simulink model "GMSK"  (R2015b)
settings: Solver=ode45  StartTime=0.0  StopTime=1000  RelTol=1e-3
undefined symbols (not defined in the file or in its folder): i
libraries: commdigbbndcpm2 x1, commrandsrc2 x1, commutil2 x1
settings Model: Creator=Алексей  LastModifiedBy=Sam
settings DataIOCC: SaveFormat=Array
settings HardwareCC: ProdBitPerPointer=32  ProdLargestAtomicFloat=None  ProdIntDivRoundTo=Undefined  ProdEndianess=Unspecified  ProdWordSize=32  ProdHWDeviceType=32-bit Generic
settings GRTTargetCC: GeneratePreprocessorConditionals=Disable all
settings ConfigComp: CovModelRefEnable=Off

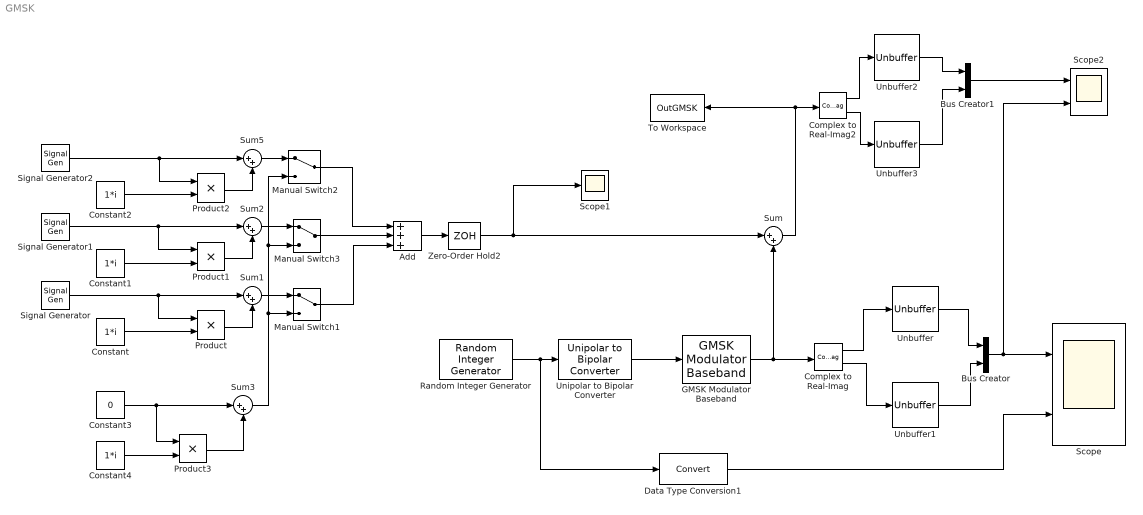
== system GMSK ==
  Add : Sum  Inputs=+++
  Bus Creator : BusCreator  Inputs=2
  Bus Creator1 : BusCreator  Inputs=2
  Complex to Real-Imag : ComplexToRealImag
  Complex to Real-Imag2 : ComplexToRealImag
  Constant{,1..2,4} (4 alike) : Constant  Value=1*i
  Constant3 : Constant  Value=0
  Data Type Conversion1 : DataTypeConversion
  GMSK Modulator Baseband : commdigbbndcpm2/GMSK Modulator Baseband  inputType=Integer  BT=.3  pulseLength=4  preHistory=1  phaseOffset=0  samplesPerSymbol=8  RateOptions=Enforce single-rate processing  outDataType=double
  Manual Switch1 : ManualSwitch
  Manual Switch2 : ManualSwitch
  Manual Switch3 : ManualSwitch
  Product{,1..3} (4 alike) : Product
  Random Integer Generator : commrandsrc2/Random Integer Generator  mul=2  seed=37  Ts=1  frameBased=off  sampPerFrame=1  orient=off  outDataType=boolean
  Scope : Scope  NumInputPorts=2
  Scope1 : Scope
  Scope2 : Scope  NumInputPorts=2
  Signal Generator : SignalGenerator  Amplitude=0.3  Frequency=100  Units=rad/sec
  Signal Generator1 : SignalGenerator  Amplitude=0.35  Frequency=1000  Units=rad/sec
  Signal Generator2 : SignalGenerator  Amplitude=0.5  Frequency=500  Units=rad/sec
  Sum{,1..3,5} (5 alike) : Sum  Inputs=|++
  To Workspace : ToWorkspace  VariableName=OutGMSK  SaveFormat=Timeseries  SampleTime=-1
      settings: Save2DSignal=2-D array (concatenate along first dimension)
  Unbuffer{,1..3} (4 alike) : Unbuffer  SampleBasedProcessing=Same as frame based
  Unipolar to Bipolar Converter : commutil2/Unipolar to Bipolar Converter  M=2  polarity=Positive  dataType=Inherit via internal rule
  Zero-Order Hold2 : ZeroOrderHold
  wires:
  Unipolar to Bipolar Converter/1 -> GMSK Modulator Baseband/1
  GMSK Modulator Baseband/1 -> Complex to Real-Imag/1, Sum/2
  Complex to Real-Imag/1 -> Unbuffer/1
  Complex to Real-Imag/2 -> Unbuffer1/1
  Unbuffer/1 -> Bus Creator/1
  Random Integer Generator/1 -> Data Type Conversion1/1, Unipolar to Bipolar Converter/1
  Bus Creator/1 -> Scope2/2, Scope/1
  Data Type Conversion1/1 -> Scope/2
  Unbuffer1/1 -> Bus Creator/2
  Signal Generator/1 -> Product/1, Sum1/1
  Complex to Real-Imag2/2 -> Unbuffer3/1
  Complex to Real-Imag2/1 -> Unbuffer2/1
  Bus Creator1/1 -> Scope2/1
  Unbuffer2/1 -> Bus Creator1/1
  Unbuffer3/1 -> Bus Creator1/2
  Product/1 -> Sum1/2
  Constant/1 -> Product/2
  Product2/1 -> Sum5/2
  Constant2/1 -> Product2/2
  Sum1/1 -> Manual Switch1/1
  Sum5/1 -> Manual Switch2/1
  Signal Generator1/1 -> Product1/1, Sum2/1
  Product1/1 -> Sum2/2
  Constant1/1 -> Product1/2
  Sum2/1 -> Manual Switch3/1
  Signal Generator2/1 -> Sum5/1, Product2/1
  Sum/1 -> To Workspace/1, Complex to Real-Imag2/1
  Manual Switch3/1 -> Add/2
  Manual Switch2/1 -> Add/1
  Manual Switch1/1 -> Add/3
  Add/1 -> Zero-Order Hold2/1
  Constant4/1 -> Product3/2
  Constant3/1 -> Product3/1, Sum3/1
  Sum3/1 -> Manual Switch1/2, Manual Switch3/2, Manual Switch2/2
  Product3/1 -> Sum3/2
  Zero-Order Hold2/1 -> Scope1/1, Sum/1
